simulink model "simulation_ex_1_2014a"  (R2014a)
settings: Solver=ode45  SolverMode=SingleTasking  StartTime=0.0  StopTime=10  RelTol=1e-3
settings Model: CovMetricSettings=dwe  CovHtmlReporting=off  covSaveCumulativeToWorkspaceVar=off  CovSaveSingleToWorkspaceVar=off  CovExternalEMLEnable=on  CovSFcnEnable=on  Creator=daiba  LastModifiedBy=HanO
settings DataIOCC: LimitDataPoints=off  SaveFormat=StructureWithTime
settings DebuggingCC: MergeDetectMultiDrivingBlocksExec=error  SolverPrmCheckMsg=none  FrameProcessingCompatibilityMsg=error  SFUnexpectedBacktrackingDiag=error  SFNoUnconditionalDefaultTransitionDiag=error
settings HardwareCC: ProdBitPerPointer=64  ProdLargestAtomicFloat=Float  ProdIntDivRoundTo=Zero  ProdEndianess=LittleEndian  ProdHWDeviceType=Specified
settings ModelReferenceCC: PropagateSignalLabelsOutOfModel=on
settings SFSimCC: SimUseLocalCustomCode=on
settings RTWCC: RTWUseLocalCustomCode=on
settings GRTTargetCC: TargetLangStandard=C99 (ISO)

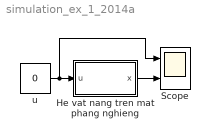
== system simulation_ex_1_2014a ==
  He vat nang tren mat phang nghieng : Subsystem  mask{m=3, alpha=pi/6, g=9.81, x_zero=0}
      mask prompts: m "Khoi luong vat nang"; alpha "Goc mat phang nghieng"; g "Gia toc trong truong"; x_zero "Vi tri ban dau"
  Scope : Scope  NumInputPorts=2
      settings: TimeRange=auto  ShowLegends=on  MaxDataPoints=5000  SaveName=ScopeData  YMin=-275.90625~-5  YMax=30.65625~5  SampleTime=-1
  u : Constant  Value=0
  wires:
  u/1 -> Scope/1, He vat nang tren mat phang nghieng/1(u)
  He vat nang tren mat phang nghieng/1(x) -> Scope/2

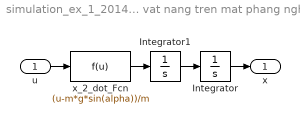
== system simulation_ex_1_2014a/He vat nang tren mat phang nghieng ==
  u : Inport
  Integrator : Integrator  InitialCondition=x_zero
  Integrator1 : Integrator
  x_2_dot_Fcn : Fcn  Expr=(u-m*g*sin(alpha))/m
  x : Outport
  wires:
  u/1 -> x_2_dot_Fcn/1
  Integrator/1 -> x/1
  x_2_dot_Fcn/1 -> Integrator1/1
  Integrator1/1 -> Integrator/1
